simulink model "Position"  (R2023b)
settings: Solver=VariableStepAuto  StartTime=0.0  StopTime=10.0  RelTol=1e-3
settings Model: Creator=Saif Mohamed  LastModifiedBy=saifg

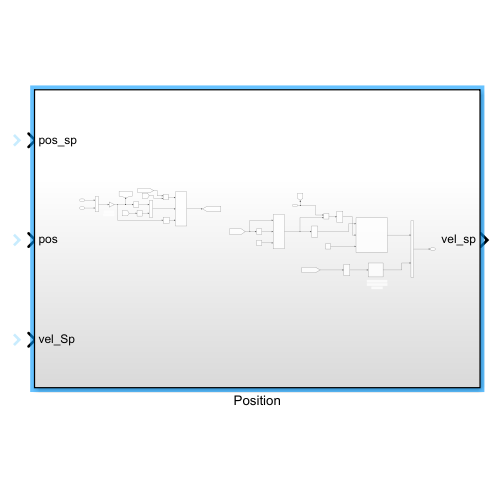
[thumbnail: Simulink's stored preview of the top-level diagram]
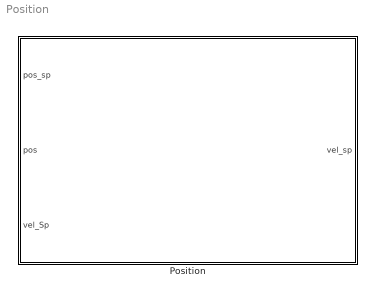
== system Position ==
  Position : Subsystem

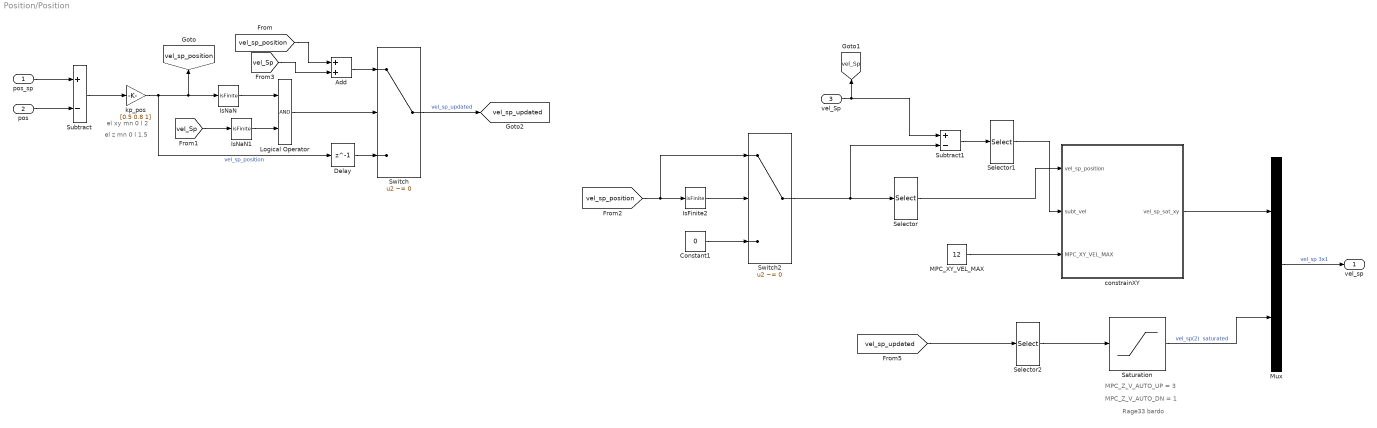
== system Position/Position ==
  note: el xy mn 0 l 2
  note: el z mn 0 l 1.5
  note: MPC_Z_V_AUTO_DN = 1
  note: MPC_Z_V_AUTO_UP = 3
  note: Rage33 bardo
  pos_sp : Inport
  pos : Inport  Port=2
  vel_Sp : Inport  Port=3
  Add : Sum
  Constant1 : Constant  Value=0
  Delay : Delay  DelayLength=1
  IsFinite2 : RelationalOperator  Operator=isFinite  OutDataTypeStr=boolean  RndMeth=Simplest  InputSameDT=off
  IsNaN : RelationalOperator  Operator=isFinite  OutDataTypeStr=boolean  RndMeth=Simplest  InputSameDT=off
  IsNaN1 : RelationalOperator  Operator=isFinite  OutDataTypeStr=boolean  RndMeth=Simplest  InputSameDT=off
  Logical Operator : Logic  AllPortsSameDT=off  OutDataTypeStr=boolean
  "MPC_XY_VEL_MAX " : Constant  Value=12
  Mux : Mux  Inputs=2
  Saturation : Saturate  UpperLimit=1  LowerLimit=-3
  Selector : Selector  InputPortWidth=3  IndexOptions=Index vector (dialog)  Indices=[1 2]  OutputSizes=1
  Selector1 : Selector  InputPortWidth=3  IndexOptions=Index vector (dialog)  Indices=[1 2]  OutputSizes=1
  Selector2 : Selector  InputPortWidth=3  IndexOptions=Index vector (dialog)  Indices=[3]  OutputSizes=1
  Subtract : Sum  Inputs=+-
  Subtract1 : Sum  Inputs=+-
  Switch : Switch  Criteria=u2 ~= 0  SaturateOnIntegerOverflow=off  InputSameDT=off
  Switch2 : Switch  Criteria=u2 ~= 0  SaturateOnIntegerOverflow=off  InputSameDT=off
  constrainXY : MATLAB Function  TreatAsAtomicUnit=on
  kp_pos : Gain  Gain=[0.5 0.8 1]
  vel_sp : Outport
  tag scope: vel_Sp=global, vel_sp_position=global, vel_sp_updated=global
  wires:
  Logical Operator/1 -> Switch/2
  IsNaN/1 -> Logical Operator/1
  kp_pos/1 -> Delay/1, [vel_sp_position], IsNaN/1  "vel_sp_position"
  Mux/1 -> vel_sp/1  "vel_sp 3x1"
  Constant1/1 -> Switch2/3
  IsFinite2/1 -> Switch2/2
  [vel_sp_position] -> Switch2/1, IsFinite2/1
  Switch/1 -> [vel_sp_updated]  "vel_sp_updated"
  Subtract1/1 -> Selector1/1
  Subtract/1 -> kp_pos/1
  [vel_Sp] -> Add/2
  Saturation/1 -> Mux/2  "vel_sp(2)  saturated"
  [vel_sp_position] -> Add/1
  Selector/1 -> constrainXY/1(vel_sp_position)
  "MPC_XY_VEL_MAX "/1 -> constrainXY/3(MPC_XY_VEL_MAX)
  Selector2/1 -> Saturation/1
  Add/1 -> Switch/1
  pos_sp/1 -> Subtract/1
  pos/1 -> Subtract/2
  Delay/1 -> Switch/3
  Switch2/1 -> Subtract1/2, Selector/1
  [vel_sp_updated] -> Selector2/1
  constrainXY/1(vel_sp_sat_xy) -> Mux/1
  [vel_Sp] -> IsNaN1/1
  Selector1/1 -> constrainXY/2(subt_vel)
  IsNaN1/1 -> Logical Operator/2
  vel_Sp/1 -> Subtract1/1, [vel_Sp]

== matlab function Position/constrainXY ==
  data: vel_sp_position input; subt_vel input; vel_sp_sat_xy output; MPC_XY_VEL_MAX input
function vel_sp_sat_xy = fcn(vel_sp_position, subt_vel, MPC_XY_VEL_MAX )

if norm( vel_sp_position + subt_vel) <= MPC_XY_VEL_MAX
    vel_sp_sat_xy = vel_sp_position+ subt_vel;

elseif norm(vel_sp_position) >= MPC_XY_VEL_MAX
    vel_sp_sat_xy = (vel_sp_position ./ norm(vel_sp_position)) .* MPC_XY_VEL_MAX;

elseif abs( norm(subt_vel - vel_sp_position) ) < 0.001
    vel_sp_sat_xy = (vel_sp_position ./ norm(vel_sp_position)) .* MPC_XY_VEL_MAX;

elseif norm(vel_sp_position) < 0.001
    vel_sp_sat_xy = (subt_vel ./ norm(subt_vel)) .* MPC_XY_VEL_MAX;

else
    u1 = subt_vel./norm(subt_vel);
    m = dot(u1, vel_sp_position);
    c = dot(vel_sp_position, vel_sp_position) - MPC_XY_VEL_MAX^2;
    s = -m + sqrt(m^2 - c);
    vel_sp_sat_xy = vel_sp_position + u1 * s;
end
